simulink model "example1_3_control"  (R2016b)
settings: Solver=VariableStepAuto  StartTime=0.0  StopTime=20  RelTol=1e-3
values from neighbouring files (symbols this model uses):
  kd = double(subs(kdsol, [wn ksi], [0.5 0.7]))    [example1_2.m]
  kp = double(subs(kpsol, [wn ksi], [0.5 0.7]))    [example1_2.m]
undefined symbols (not defined in the file or in its folder): A, B, C
settings Model: Creator=Trancemania  LastModifiedBy=Trancemania

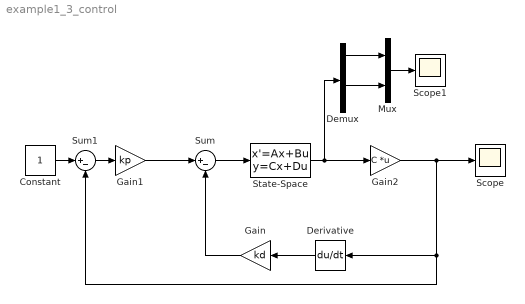
== system example1_3_control ==
  Constant : Constant
  Demux : Demux
  Derivative : Derivative
  Gain : Gain  Gain=kd
  Gain1 : Gain  Gain=kp
  Gain2 : Gain  Gain=C  Multiplication=Matrix(K*u)
  Mux : Mux  Inputs=2
  Scope : Scope
  Scope1 : Scope
  State-Space : StateSpace  A=A  B=B  C=eye(4)  D=zeros(4,1)  X0=0
  Sum : Sum  Inputs=|+-
  Sum1 : Sum  Inputs=|+-
  wires:
  Gain2/1 -> Scope/1, Sum1/2, Derivative/1
  Constant/1 -> Sum1/1
  Derivative/1 -> Gain/1
  Gain1/1 -> Sum/1
  Gain/1 -> Sum/2
  Sum1/1 -> Gain1/1
  State-Space/1 -> Demux/1, Gain2/1
  Demux/1 -> Mux/1
  Demux/3 -> Mux/2
  Mux/1 -> Scope1/1
  Sum/1 -> State-Space/1
